simulink model "Binary_search_tightening"  (R2023b)
settings: Solver=FixedStepAuto  StartTime=0.0  StopTime=30  FixedStep=1e-3  RelTol=1e-3
libraries: arduinolib x3, dspfdesign x2, slpidlib x1
settings Model: Creator=doria  LastModifiedBy=doria

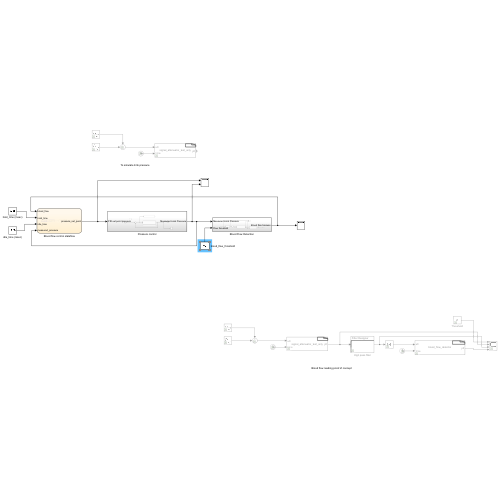
[thumbnail: Simulink's stored preview of the top-level diagram]
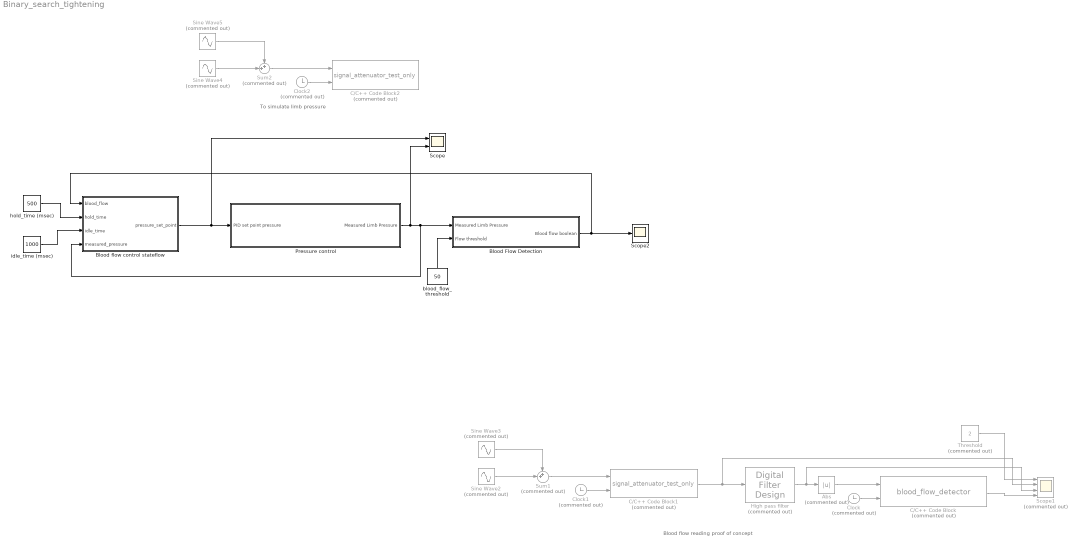
== system Binary_search_tightening ==
  note: To simulate limb pressure
  note: Blood flow reading proof of concept
  Abs : Abs  Commented=on  SaturateOnIntegerOverflow=off
  Blood Flow Detection : Subsystem
  Blood flow control stateflow : Stateflow chart  TreatAsAtomicUnit=on
  C/C++ Code Block : S-Function  Commented=on  FunctionName=blood_flow_detector  SFunctionModules=blood_flow_detector_wrapper.c  SFunctionDeploymentMode=off  EnableBusSupport=off  mask(S-Function Builder){}
      mask help: Simulink:masks:SFunctionBuilder_MD
      mask init:
      | val = [[.9  0.75 0.75 1 1 .9 .9 1]',[1 1 0.75 0.75 .9 .9 1 .9]'];try , sys = get_param(gcb,'SfunBuilderFcnName');if isempty(sys), sys = get_param(gcb,'FunctionName'); end,catch, sys = get_param(gcb,'FunctionName'); end
      settings: CopyFcn=set_param(gcbh,'LinkStatus','none')  OpenFcn=sfunctionwizard(gcbh)
      mask Display:
      | plot(val(:,1),val(:,2))
      | disp(sys)
      | port_label('input',1,'u0')
      | port_label('input',2,'time')
      | port_label('output',1,'y0')
  C/C++ Code Block1 : S-Function  Commented=on  FunctionName=signal_attenuator_test_only  SFunctionModules=signal_attenuator_test_only_wrapper.c  SFunctionDeploymentMode=off  EnableBusSupport=off  mask(S-Function Builder){}
      mask help: Simulink:masks:SFunctionBuilder_MD
      mask init: same as Binary_search_tightening/C/C++ Code Block
      settings: CopyFcn=set_param(gcbh,'LinkStatus','none')  OpenFcn=sfunctionwizard(gcbh)
      mask Display:
      | plot(val(:,1),val(:,2))
      | disp(sys)
      | port_label('input',1,'u0')
      | port_label('input',2,'time')
      | port_label('output',1,'y0')
  C/C++ Code Block2 : S-Function  Commented=on  FunctionName=signal_attenuator_test_only  SFunctionModules=signal_attenuator_test_only_wrapper.c  SFunctionDeploymentMode=off  EnableBusSupport=off  mask(S-Function Builder){}
      mask help: Simulink:masks:SFunctionBuilder_MD
      mask init: same as Binary_search_tightening/C/C++ Code Block
      settings: CopyFcn=set_param(gcbh,'LinkStatus','none')  OpenFcn=sfunctionwizard(gcbh)
      mask Display:
      | plot(val(:,1),val(:,2))
      | disp(sys)
      | port_label('input',1,'u0')
      | port_label('input',2,'time')
      | port_label('output',1,'y0')
  Clock : Clock  Commented=on
  Clock1 : Clock  Commented=on
  Clock2 : Clock  Commented=on
  High pass filter : dspfdesign/Digital Filter Design  Commented=on  mwdsp_browser_bugfix_var=off
  Pressure control : Subsystem
  Scope : Scope  NumInputPorts=2
  Scope1 : Scope  Commented=on  NumInputPorts=4
  Scope2 : Scope
  Sine Wave2 : Sin  Commented=on  Amplitude=0.1  Frequency=50  SampleTime=0
  Sine Wave3 : Sin  Commented=on  SampleTime=0
  Sine Wave4 : Sin  Commented=on  Amplitude=0.1  Frequency=50  SampleTime=0
  Sine Wave5 : Sin  Commented=on  SampleTime=0
  Sum1 : Sum  Commented=on  Inputs=++|
  Sum2 : Sum  Commented=on  Inputs=++|
  Threshold : Constant  Commented=on  Value=2
  blood_flow_threshold : Constant  Value=50
  hold_time (msec) : Constant  Value=500
  idle_time (msec) : Constant  Value=1000
  wires:
  Sine Wave3/1 -> Sum1/1
  Sine Wave2/1 -> Sum1/2
  Sum1/1 -> C/C++ Code Block1/1
  Abs/1 -> C/C++ Code Block/1
  Clock/1 -> C/C++ Code Block/2
  Clock1/1 -> C/C++ Code Block1/2
  C/C++ Code Block/1 -> Scope1/4
  High pass filter/1 -> Scope1/3, Abs/1
  Threshold/1 -> Scope1/1
  C/C++ Code Block1/1 -> Scope1/2, High pass filter/1
  blood_flow_threshold/1 -> Blood Flow Detection/2(Flow threshold)
  Clock2/1 -> C/C++ Code Block2/2
  Sum2/1 -> C/C++ Code Block2/1
  Sine Wave4/1 -> Sum2/2
  Sine Wave5/1 -> Sum2/1
  Blood flow control stateflow/1(pressure_set_point) -> Scope/1, Pressure control/1(PID set point pressure)
  Blood Flow Detection/1(Blood flow boolean) -> Blood flow control stateflow/1(blood_flow), Scope2/1
  hold_time (msec)/1 -> Blood flow control stateflow/2(hold_time)
  idle_time (msec)/1 -> Blood flow control stateflow/3(idle_time)
  Pressure control/1(Measured Limb Pressure) -> Blood flow control stateflow/4(measured_pressure), Blood Flow Detection/1(Measured Limb Pressure), Scope/2

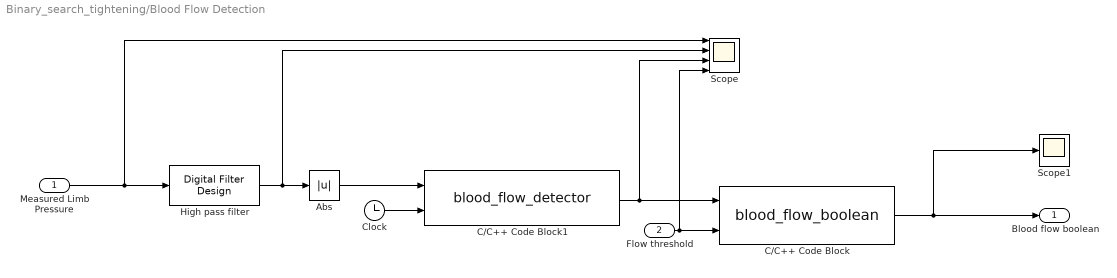
== system Binary_search_tightening/Blood Flow Detection ==
  Measured Limb Pressure : Inport
  Flow threshold : Inport  Port=2
  Abs : Abs  SaturateOnIntegerOverflow=off
  C/C++ Code Block : S-Function  FunctionName=blood_flow_boolean  SFunctionModules=blood_flow_boolean_wrapper.c  SFunctionDeploymentMode=off  EnableBusSupport=off  mask(S-Function Builder){}
      mask help: Simulink:masks:SFunctionBuilder_MD
      mask init: same as Binary_search_tightening/C/C++ Code Block
      settings: CopyFcn=set_param(gcbh,'LinkStatus','none')  OpenFcn=sfunctionwizard(gcbh)
      mask Display:
      | plot(val(:,1),val(:,2))
      | disp(sys)
      | port_label('input',1,'blood_flow')
      | port_label('input',2,'flow_thresh')
      | port_label('output',1,'y0')
  C/C++ Code Block1 : S-Function  FunctionName=blood_flow_detector  SFunctionModules=blood_flow_detector_wrapper.c  SFunctionDeploymentMode=off  EnableBusSupport=off  mask(S-Function Builder){}
      mask help: Simulink:masks:SFunctionBuilder_MD
      mask init: same as Binary_search_tightening/C/C++ Code Block
      settings: CopyFcn=set_param(gcbh,'LinkStatus','none')  OpenFcn=sfunctionwizard(gcbh)
      mask Display:
      | plot(val(:,1),val(:,2))
      | disp(sys)
      | port_label('input',1,'u0')
      | port_label('input',2,'time')
      | port_label('output',1,'y0')
  Clock : Clock
  High pass filter : dspfdesign/Digital Filter Design  mwdsp_browser_bugfix_var=off
  Scope : Scope  NumInputPorts=4
  Scope1 : Scope
  Blood flow boolean : Outport
  wires:
  C/C++ Code Block/1 -> Scope1/1, Blood flow boolean/1
  Abs/1 -> C/C++ Code Block1/1
  Clock/1 -> C/C++ Code Block1/2
  Measured Limb Pressure/1 -> Scope/1, High pass filter/1
  High pass filter/1 -> Scope/2, Abs/1
  C/C++ Code Block1/1 -> Scope/3, C/C++ Code Block/1
  Flow threshold/1 -> Scope/4, C/C++ Code Block/2

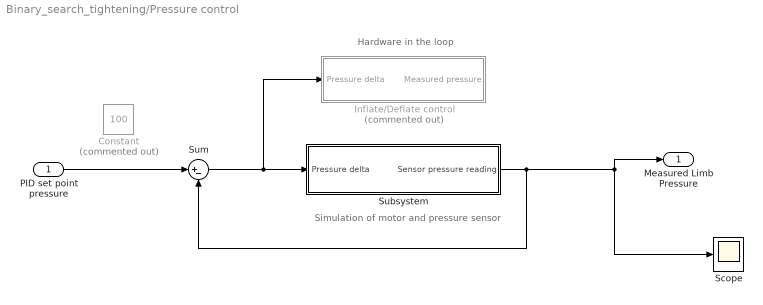
== system Binary_search_tightening/Pressure control ==
  note: Simulation of motor and pressure sensor
  note: Hardware in the loop
  PID set point pressure : Inport
  Constant : Constant  Commented=on  Value=100
  Inflate/Deflate control : Subsystem  Commented=on
  Scope : Scope
  Subsystem : Subsystem
  Sum : Sum  Inputs=|+-
  Measured Limb Pressure : Outport
  wires:
  Sum/1 -> Subsystem/1(Pressure delta), Inflate/Deflate control/1(Pressure delta)
  Subsystem/1(Sensor pressure reading) -> Measured Limb Pressure/1, Scope/1, Sum/2
  PID set point pressure/1 -> Sum/1

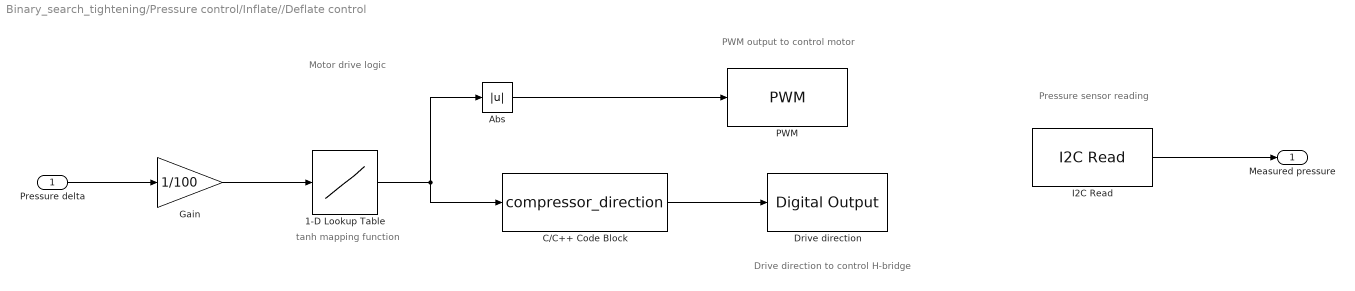
== system Binary_search_tightening/Pressure control/Inflate//Deflate control ==
  note: Pressure sensor reading
  note: Motor drive logic
  note: Drive direction to control H-bridge
  note: PWM output to control motor
  note: tanh mapping function
  Pressure delta : Inport
  1-D Lookup Table : Lookup_n-D  NumberOfTableDimensions=1  BreakpointsForDimension1=[-5:5]  Table=tanh([-5:5])  InternalRulePriority=Speed  RndMeth=Simplest
  Abs : Abs  SaturateOnIntegerOverflow=off
  C/C++ Code Block : S-Function  FunctionName=compressor_direction  SFunctionModules=compressor_direction_wrapper.c  SFunctionDeploymentMode=off  EnableBusSupport=off  mask(S-Function Builder){}
      mask help: Simulink:masks:SFunctionBuilder_MD
      mask init: same as Binary_search_tightening/C/C++ Code Block
      settings: CopyFcn=set_param(gcbh,'LinkStatus','none')  OpenFcn=sfunctionwizard(gcbh)
      mask Display:
      | plot(val(:,1),val(:,2))
      | disp(sys)
      | port_label('input',1,'u0')
      | port_label('output',1,'y0')
  Drive direction : arduinolib/Digital Output  pinNumber=9  Direction=output  blockPlatform=arduino
  Gain : Gain  Gain=1/100
  I2C Read : arduinolib/I2C Read  I2CModule=0  Mode=Master  SlaveAddress=10  SlaveByteOrder=BigEndian  Direction=Receiver  RegisterAddressMode=on  RegisterAddress=0  SlaveDataType=uint8  DataLength=1  NoAck=off  RepeatedStart=off  OutputStatus=off  blockPlatform=ARDUINO  SampleTime=0.1
  PWM : arduinolib/PWM  pinNumber=5  frequencyType=Default  desiredFrequency=490.2  achievableFrequency=490.2
  Measured pressure : Outport
  wires:
  Pressure delta/1 -> Gain/1
  Gain/1 -> 1-D Lookup Table/1
  1-D Lookup Table/1 -> C/C++ Code Block/1, Abs/1
  Abs/1 -> PWM/1
  C/C++ Code Block/1 -> Drive direction/1
  I2C Read/1 -> Measured pressure/1

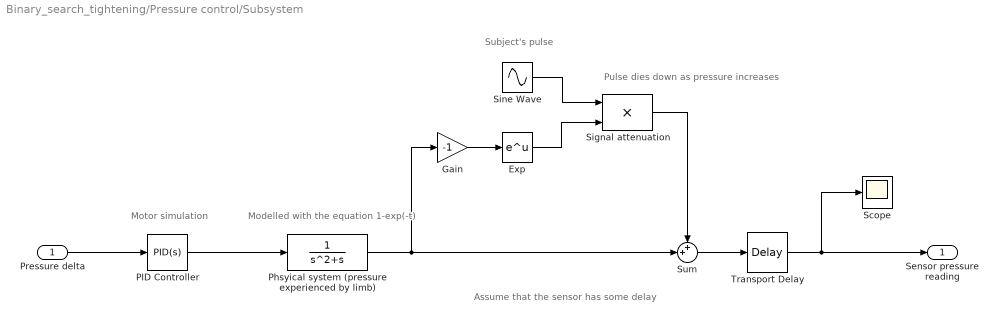
== system Binary_search_tightening/Pressure control/Subsystem ==
  note: Pulse dies down as pressure increases
  note: Subject's pulse
  note: Motor simulation
  note: Assume that the sensor has some delay
  note: Modelled with the equation 1-exp(-t)
  Pressure delta : Inport
  Exp : Math
  Gain : Gain  Gain=-1
  PID Controller : slpidlib/PID Controller  Controller=PID  Form=Parallel  TimeDomain=Continuous-time  UseExternalTs=off  SampleTime=-1  IntegratorMethod=Forward Euler  FilterMethod=Forward Euler  ControllerParametersSource=internal  P=2  I=3  UseKiTs=off  D=7  N=100  UseFilter=on  TunerSelectOption=Transfer Function Based (PID Tuner App)  InitialConditionSource=internal  InitialConditionForIntegrator=0  InitialConditionForFilter=0  DifferentiatorICPrevScaledInput=0  ExternalReset=none  TrackingMode=off  Kt=1  LimitOutput=off  SatLimitsSource=internal  UpperSaturationLimit=inf  LowerSaturationLimit=-inf  LinearizeAsGain=on  AntiWindupMode=none  Kb=1  LimitIntegrator=off  UpperIntegratorSaturationLimit=inf  LowerIntegratorSaturationLimit=-inf  POutMin=[]  POutMax=[]  IOutMin=[]  IOutMax=[]  DOutMin=[]  DOutMax=[]  NOutMin=[]  NOutMax=[]  SumOutMin=[]  SumOutMax=[]  SaturationOutMin=[]  SaturationOutMax=[]  PParamMin=[]  PParamMax=[]  IParamMin=[]  IParamMax=[]  DParamMin=[]  DParamMax=[]  NParamMin=[]  NParamMax=[]  KbParamMin=[]  KbParamMax=[]  KtParamMin=[]  KtParamMax=[]  KbOutMin=[]  KbOutMax=[]  KtOutMin=[]  KtOutMax=[]  IntegratorOutMin=[]  IntegratorOutMax=[]  FilterOutMin=[]  FilterOutMax=[]  SumI1OutMin=[]  SumI1OutMax=[]  SumI2OutMin=[]  SumI2OutMax=[]  SumI3OutMin=[]  SumI3OutMax=[]  SumI4OutMin=[]  SumI4OutMax=[]  SumDOutMin=[]  SumDOutMax=[]  DifferentiatorOutMin=[]  DifferentiatorOutMax=[]  FilterDiffOutCoefMin=[]  FilterDiffOutCoefMax=[]  ReciprocalOutMin=[]  ReciprocalOutMax=[]  SumDenOutMin=[]  SumDenOutMax=[]  SumNumOutMin=[]  SumNumOutMax=[]  DivideOutMin=[]  DivideOutMax=[]  UdiffTsProdOutMin=[]  UdiffTsProdOutMax=[]  NTsProdOutMin=[]  NTsProdOutMax=[]  UintegralTsProdOutMin=[]  UintegralTsProdOutMax=[]  UngainTsProdOutMin=[]  UngainTsProdOutMax=[]  ClampingZeroOutDataTypeStr=Inherit: Inherit via back propagation  ClampingZeroOutMin=[]  ClampingZeroOutMax=[]  FilterDenConstantOutDataTypeStr=Inherit: Inherit via back propagation  FilterDenConstantOutMin=[]  FilterDenConstantOutMax=[]  PCopyOutDataTypeStr=Inherit: Inherit via back propagation  PCopyOutMin=[]  PCopyOutMax=[]  NCopyOutDataTypeStr=Inherit: Inherit via back propagation  NCopyOutMin=[]  NCopyOutMax=[]  IntegratorContinuousStateAttributes=''  IntegratorStateMustResolveToSignalObject=off  IntegratorRTWStateStorageClass=Auto  FilterContinuousStateAttributes=''  FilterStateMustResolveToSignalObject=off  FilterRTWStateStorageClass=Auto  ParallelPVariant=InternalParameters  IdealPVariant=Disabled  IVariant=InternalParameters  DVariant=InternalParameters  IntegratorVariant=Continuous  SatVariant=Disabled  AWVariant=Passthrough  PCopyVariant=Disabled  TRVariant=Disabled  FdbkBlocksVariant=Forward  IdealPFdbkVariant=Disabled  SatFdbkVariant=Disabled  DerivativeFilterVariant=ContFilter  NVariant=InternalParameters  NCopyVariant=Disabled  FilterICVariant=InternalICsFilter  IntegratorICVariant=InternalICs  ExternalResetVariant=Disabled  TRSumVariant=Passthrough  SumFdbkVariant=Disabled  SumVariant=Sum_PID  TsampFilterVariant=InternalTs  TsampNgainVariant=Passthrough  TsampIntegralVariant=Disabled_SignalSpec  ExternalSaturationOutDataTypeStr=Inherit: Same as second input
  Phsyical system (pressure experienced by limb) : TransferFcn  Denominator=[1 1 0]
  Scope : Scope
  Signal attenuation : Product  Inputs=**
  Sine Wave : Sin  Amplitude=10  Frequency=50  SampleTime=0
  Sum : Sum  Inputs=++|
  Transport Delay : TransportDelay  DelayTime=0.1
  Sensor pressure reading : Outport
  wires:
  PID Controller/1 -> Phsyical system (pressure experienced by limb)/1
  Transport Delay/1 -> Scope/1, Sensor pressure reading/1
  Pressure delta/1 -> PID Controller/1
  Phsyical system (pressure experienced by limb)/1 -> Sum/2, Gain/1
  Sum/1 -> Transport Delay/1
  Sine Wave/1 -> Signal attenuation/1
  Signal attenuation/1 -> Sum/1
  Exp/1 -> Signal attenuation/2
  Gain/1 -> Exp/1

== stateflow chart Binary_search_tightening/Blood flow control stateflow ==
  state Binary_search_ideal_pressure
    % Find ideal pressure to stop bleeding between pressure extremes measured in previous stage
    entry:
    binary_search_upper = pressure_upper_bound
    binary_search_lower = pressure_lower_bound
    ideal_pressure_found = 0
    state Too_tight
      entry:
      binary_search_upper = pressure_set_point
    state Adjust_pressure_set_point
      entry:
      pressure_set_point = (binary_search_upper + binary_search_lower)/2
      pressure_difference = binary_search_upper - binary_search_lower
    state Ideal_pressure_found
      entry:
      pressure_set_point = binary_search_upper
      ideal_pressure_found = 1
    state Too_loose
      entry:
      binary_search_lower = pressure_set_point
    Too_tight -> Adjust_pressure_set_point
    (junction 48) -> Too_tight [order 2] : [pressure_difference >= 25 && blood_flow == 0]
    (default) -> Adjust_pressure_set_point
    Adjust_pressure_set_point -> (junction 48) : after(hold_time, msec)[pressure_set_point == measured_pressure]
    (junction 48) -> Ideal_pressure_found [order 1] : [pressure_difference < 25]
    (junction 48) -> Too_loose [order 3] : [pressure_difference >= 25 && blood_flow > 0]
    Too_loose -> Adjust_pressure_set_point
  state Find_initial_bounds
    entry:
    pressure_set_point = 100
    upper_bound_found = 0
    state Inflate
      %Inflate quickly to stop blood flow
      exit:
      pressure_upper_bound = pressure_set_point
      state Increase_pressure_set_point
        entry:
        pressure_set_point = pressure_set_point + 10
      state wait
      wait -> Increase_pressure_set_point : [measured_pressure >= pressure_set_point]
      Increase_pressure_set_point -> wait
      (default) -> wait
    state Deflate
      % Slowly deflate until blood flow returns
      exit:
      pressure_lower_bound = pressure_set_point
      state Decrease_pressure_set_point
        entry:
        pressure_set_point = pressure_set_point - 5
      state Wait
      (default) -> Decrease_pressure_set_point
      Wait -> Decrease_pressure_set_point : [measured_pressure<pressure_set_point]
      Decrease_pressure_set_point -> Wait
    (default) -> Inflate
    Inflate -> Deflate : after(hold_time,msec)[blood_flow == 0]{upper_bound_found = 1}
  state Fine_adjustments
    state Increase_pressure
      entry:
      pressure_set_point = pressure_set_point + 5
    state Default_state
    state Decrease_pressure
      entry:
      pressure_set_point = pressure_set_point - 1
    (junction 64) -> Increase_pressure [order 1] : [blood_flow>0]
    (default) -> Default_state
    Increase_pressure -> (junction 76)
    Default_state -> (junction 64)
    (junction 76) -> (junction 64) : after(hold_time,msec)
    (junction 64) -> Decrease_pressure [order 2] : [blood_flow ==0]
    Decrease_pressure -> (junction 76)
  state Idle
    % Wait in the idle state for a given amount of time
  (default) -> Find_initial_bounds
  Fine_adjustments -> Idle : after(hold_time*5,msec)[blood_flow == 0]
  Binary_search_ideal_pressure -> Idle : [ideal_pressure_found==1]
  Idle -> (junction 59) : after(idle_time,msec)
  (junction 59) -> Fine_adjustments [order 1] : [blood_flow > 0]
  Find_initial_bounds -> Binary_search_ideal_pressure : after(hold_time,msec)[blood_flow>0 && upper_bound_found == true]
  (junction 59) -> Idle [order 2] : [blood_flow == 0]
  data: pressure_set_point output double; blood_flow input; hold_time input; idle_time input; measured_pressure input; binary_search_lower local; binary_search_upper local; ideal_pressure_found local; pressure_difference local; pressure_lower_bound local; pressure_upper_bound local; upper_bound_found local
